simulink model "Flowchart8"  (Simulink 6.0)
settings: Solver=ode45  StartTime=0.0  StopTime=10.0  RelTol=1e-3
settings Model: Creator=scaife  LastModifiedBy=scaife  ExtModeAutoUpdateStatusClock=off
settings DataIOCC: SignalLoggingName=sigsOut
settings DebuggingCC: SolverPrmCheckMsg=none
settings HardwareCC: TargetUnknown=on
settings GRTTargetCC: ModelReferenceCompliant=off  MatFileLogging=off

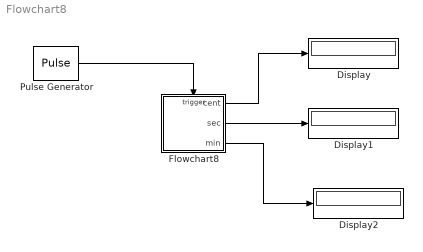
== system Flowchart8 ==
  Display : Display
  Display1 : Display
  Display2 : Display
  Flowchart8 : Stateflow chart
  Pulse Generator : DiscretePulseGenerator
  wires:
  Pulse Generator/1 -> Flowchart8/Trigger
  Flowchart8/1(cent) -> Display/1
  Flowchart8/2(sec) -> Display1/1
  Flowchart8/3(min) -> Display2/1

== stateflow chart Flowchart8 ==
  state A
  (junction 5) -> (junction 6) : [sec==3]{sec=0; min++}
  A -> (junction 4) : TIC{cent++}
  (junction 4) -> (junction 5) : [cent==2]{cent=0; sec++}
  (junction 4) -> (junction 6)
  (junction 5) -> (junction 6)
  (default) -> A
  data: cent output int32; sec output int32; min output int32
  events: TIC input EITHER_EDGE_EVENT
